simulink model "VAB_non_linear"  (R2019b)
settings: Solver=VariableStepAuto  StartTime=0.0  StopTime=t_end  FixedStep=Ts  RelTol=1e-3
undefined symbols (not defined in the file or in its folder): control_on, J_m_star, k_simulazione_continua, k_t, L, m_c_simulazione, phi_iniziale, phi_p_iniziale, phi_p_setpoint, phi_secondo, R, theta_iniziale, theta_p_iniziale, theta_secondo
libraries: cstblocks x1
settings Model: Creator=miche  LastModifiedBy=AndreaCalegari

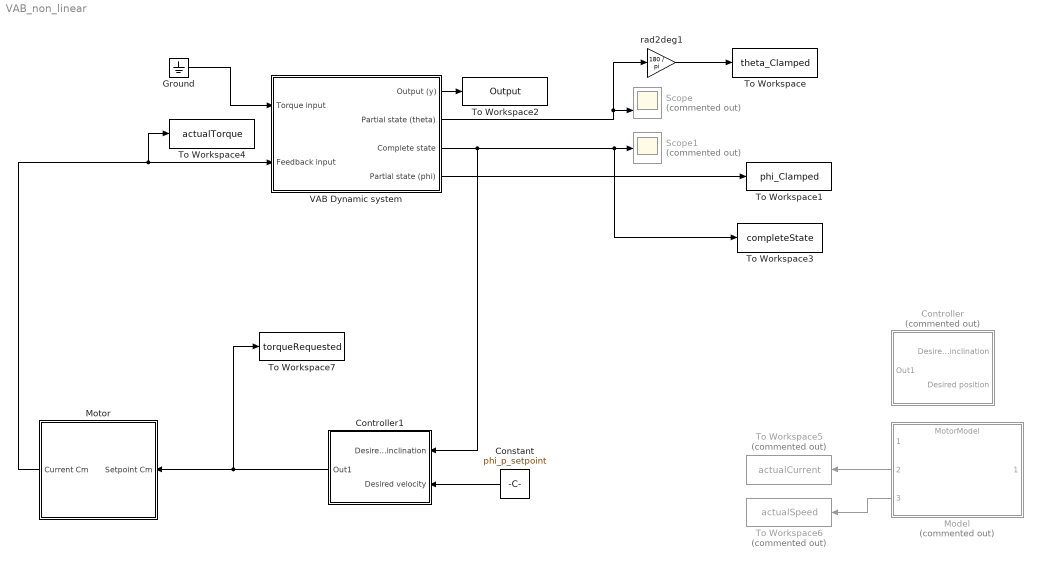
== system VAB_non_linear ==
  Constant : Constant  Value=phi_p_setpoint
  Controller : Subsystem  Commented=on
  Controller1 : Subsystem
  Ground : Ground
  Model : ModelReference  Commented=on  ModelNameDialog=MotorModel.slx  SimulationMode=Normal  ModelReferenceVersion=1.9
  "Motor " : Subsystem
  Scope : Scope  Commented=on  NumInputPorts=2
  Scope1 : Scope  Commented=on
  To Workspace : ToWorkspace  VariableName=theta_Clamped  SampleTime=-1
  To Workspace1 : ToWorkspace  VariableName=phi_Clamped  SampleTime=-1
  To Workspace2 : ToWorkspace  VariableName=Output  SampleTime=-1
  To Workspace3 : ToWorkspace  VariableName=completeState  SampleTime=-1
  To Workspace4 : ToWorkspace  VariableName=actualTorque  SampleTime=-1
  To Workspace5 : ToWorkspace  Commented=on  VariableName=actualCurrent  SampleTime=-1
  To Workspace6 : ToWorkspace  Commented=on  VariableName=actualSpeed  SampleTime=-1
  To Workspace7 : ToWorkspace  VariableName=torqueRequested  SampleTime=-1
  VAB Dynamic system : Subsystem
  rad2deg1 : Gain  Gain=180 / pi
  wires:
  VAB Dynamic system/2(Partial state (theta)) -> rad2deg1/1, Scope/2
  VAB Dynamic system/1(Output (y)) -> To Workspace2/1
  Ground/1 -> VAB Dynamic system/1(Torque input)
  VAB Dynamic system/3("Complete state ") -> Controller1/1(Desired inclination), To Workspace3/1, Scope1/1
  rad2deg1/1 -> To Workspace/1
  VAB Dynamic system/4(Partial state (phi)) -> To Workspace1/1
  Model/3 -> To Workspace6/1
  Model/2 -> To Workspace5/1
  Controller1/1(Out1) -> To Workspace7/1, "Motor "/1(Setpoint Cm)
  "Motor "/1("Current Cm ") -> To Workspace4/1, VAB Dynamic system/2(Feedback input)
  Constant/1 -> Controller1/2("Desired velocity ")

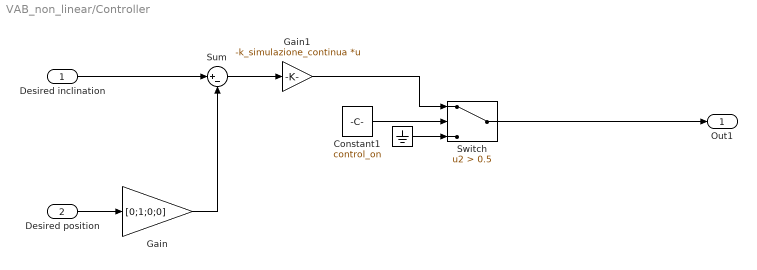
== system VAB_non_linear/Controller ==
  Desired inclination : Inport
  "Desired position " : Inport  Port=2
  " " : Ground
  Constant1 : Constant  Value=control_on
  Gain : Gain  Gain=[0;1;0;0]
  Gain1 : Gain  Gain=-k_simulazione_continua  Multiplication=Matrix(K*u)
  Sum : Sum  Inputs=|+-
  Switch : Switch  Criteria=u2 > Threshold  Threshold=0.5
  Out1 : Outport
  wires:
  Constant1/1 -> Switch/2
  " "/1 -> Switch/3
  Sum/1 -> Gain1/1
  Desired inclination/1 -> Sum/1
  Gain/1 -> Sum/2
  "Desired position "/1 -> Gain/1
  Gain1/1 -> Switch/1
  Switch/1 -> Out1/1

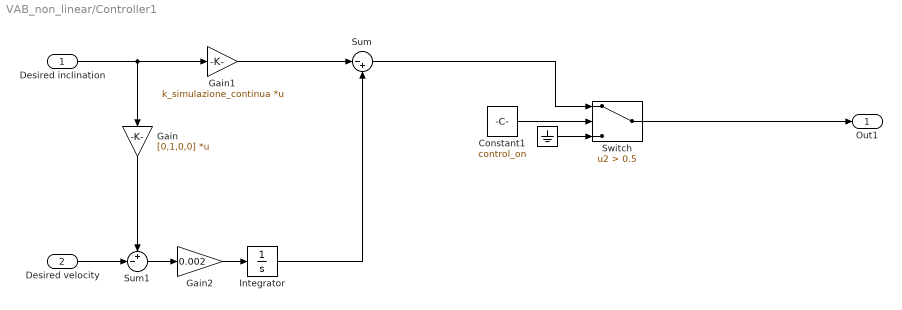
== system VAB_non_linear/Controller1 ==
  Desired inclination : Inport
  "Desired velocity " : Inport  Port=2
  " " : Ground
  Constant1 : Constant  Value=control_on
  Gain : Gain  Gain=[0,1,0,0]  Multiplication=Matrix(K*u)
  Gain1 : Gain  Gain=k_simulazione_continua  Multiplication=Matrix(K*u)
  Gain2 : Gain  Gain=0.002
  Integrator : Integrator
  Sum : Sum  Inputs=|-+
  Sum1 : Sum  Inputs=+-|
  Switch : Switch  Criteria=u2 > Threshold  Threshold=0.5
  Out1 : Outport
  wires:
  Switch/1 -> Out1/1
  Constant1/1 -> Switch/2
  " "/1 -> Switch/3
  Desired inclination/1 -> Gain1/1, Gain/1
  Gain/1 -> Sum1/1
  "Desired velocity "/1 -> Sum1/2
  Sum1/1 -> Gain2/1
  Gain1/1 -> Sum/1
  Integrator/1 -> Sum/2
  Sum/1 -> Switch/1
  Gain2/1 -> Integrator/1

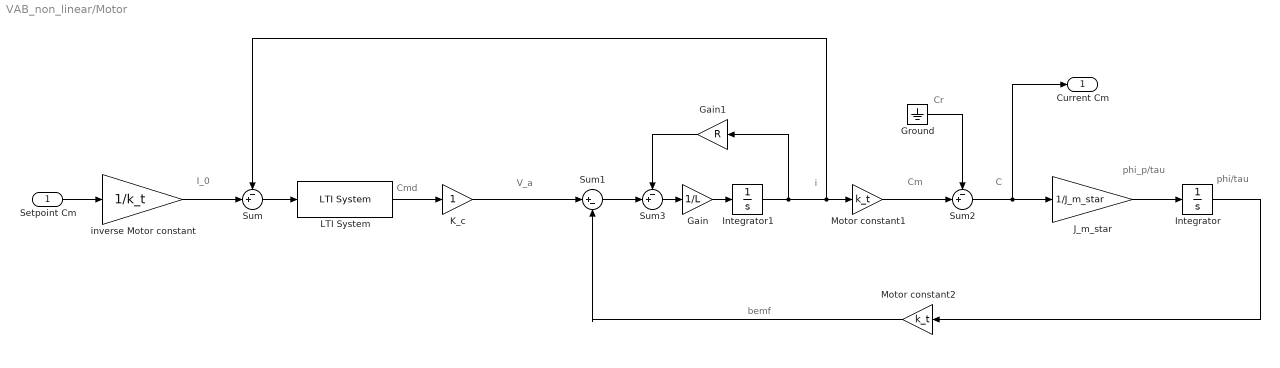
== system VAB_non_linear/Motor  ==
  note: bemf
  note: phi/tau
  note: phi_p/tau
  note: C
  note: i
  note: Cmd
  note: V_a
  note: I_0
  note: Cm
  note: Cr
  Setpoint Cm : Inport
  Gain : Gain  Gain=1/L
  Gain1 : Gain  Gain=R
  Ground : Ground
  Integrator : Integrator
  Integrator1 : Integrator
  "J_m_star " : Gain  Gain=1/J_m_star
  K_c : Gain
  LTI System : cstblocks/LTI System  sys=PI_I  IC=[]
  Motor constant1 : Gain  Gain=k_t
  Motor constant2 : Gain  Gain=k_t
  Sum : Sum  Inputs=-+|
  Sum1 : Sum  Inputs=|+-
  Sum2 : Sum  Inputs=-+|
  Sum3 : Sum  Inputs=-+|
  inverse Motor constant : Gain  Gain=1/k_t
  "Current Cm " : Outport
  wires:
  Integrator/1 -> Motor constant2/1
  Motor constant1/1 -> Sum2/2
  K_c/1 -> Sum1/1
  Integrator1/1 -> Gain1/1, Sum/1, Motor constant1/1
  inverse Motor constant/1 -> Sum/2
  Sum2/1 -> "Current Cm "/1, "J_m_star "/1
  "J_m_star "/1 -> Integrator/1
  Ground/1 -> Sum2/1
  Motor constant2/1 -> Sum1/2
  Setpoint Cm/1 -> inverse Motor constant/1
  Gain/1 -> Integrator1/1
  Sum3/1 -> Gain/1
  Sum1/1 -> Sum3/2
  Gain1/1 -> Sum3/1
  Sum/1 -> LTI System/1
  LTI System/1 -> K_c/1

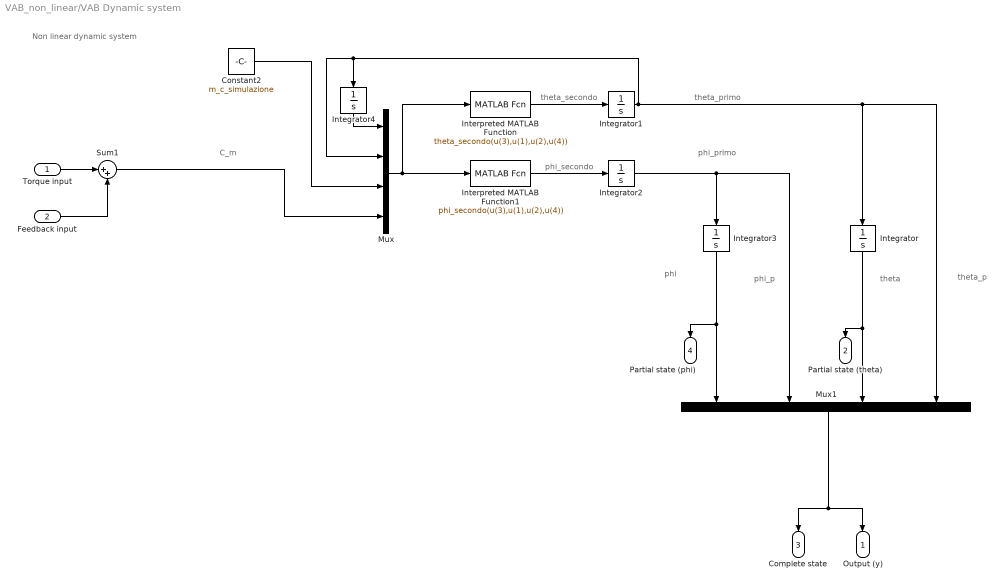
== system VAB_non_linear/VAB Dynamic system ==
  note: Non linear dynamic system
  note: phi_primo
  note: phi
  note: theta_p
  note: theta
  note: phi_p
  note: phi_secondo
  note: C_m
  note: theta_secondo
  note: theta_primo
  Torque input : Inport
  Feedback input : Inport  Port=2
  Constant2 : Constant  Value=m_c_simulazione
  Integrator : Integrator  InitialCondition=theta_iniziale
  Integrator1 : Integrator  InitialCondition=theta_p_iniziale  UpperSaturationLimit=100  LowerSaturationLimit=-100
  Integrator2 : Integrator  InitialCondition=phi_p_iniziale
  Integrator3 : Integrator  InitialCondition=phi_iniziale
  Integrator4 : Integrator  InitialCondition=theta_iniziale
  Interpreted MATLAB Function : MATLABFcn  MATLABFcn=theta_secondo(u(3),u(1),u(2),u(4))  OutputDimensions=1
  Interpreted MATLAB Function1 : MATLABFcn  MATLABFcn=phi_secondo(u(3),u(1),u(2),u(4))
  Mux : Mux
  Mux1 : Mux
  Sum1 : Sum  Inputs=|++
  Output (y) : Outport
  Partial state (theta) : Outport  Port=2
  "Complete state " : Outport  Port=3
  Partial state (phi) : Outport  Port=4
  wires:
  Feedback input/1 -> Sum1/2
  Torque input/1 -> Sum1/1
  Integrator3/1 -> Partial state (phi)/1, Mux1/1
  Constant2/1 -> Mux/3
  Sum1/1 -> Mux/4
  Integrator4/1 -> Mux/1
  Interpreted MATLAB Function1/1 -> Integrator2/1
  Integrator2/1 -> Mux1/2, Integrator3/1
  Integrator1/1 -> Integrator4/1, Mux/2, Mux1/4, Integrator/1
  Integrator/1 -> Partial state (theta)/1, Mux1/3
  Interpreted MATLAB Function/1 -> Integrator1/1
  Mux1/1 -> Output (y)/1, "Complete state "/1
  Mux/1 -> Interpreted MATLAB Function/1, Interpreted MATLAB Function1/1
